simulink model "BallAndPlate_system"  (R2024a)
settings: Solver=ode23t  StartTime=0.0  StopTime=StopTime  RelTol=1e-3  AbsTol=1e-3
settings Model: DataDictionary=BallAndPlate_system_data.sldd  Creator=tshintai  LastModifiedBy=tshintai
settings SolverCC: AutoScaleAbsTol=off  DaesscMode=Fast
settings OptimizationCC: DefaultParameterBehavior=Inlined  EnhancedBackFolding=on  PassReuseOutputArgsAs=Individual arguments  ZeroExternalMemoryAtStartup=off  ZeroInternalMemoryAtStartup=off  OptimizeBlockOrder=speed  DifferentSizesBufferReuse=on  OptimizationCustomize=off  EfficientTunableParamExpr=on
settings DebuggingCC: ParameterPrecisionLossMsg=none  ParameterTunabilityLossMsg=error  UnconnectedInputMsg=warning  UnconnectedOutputMsg=warning  UnconnectedLineMsg=warning
settings ModelReferenceCC: EnableRefExpFcnMdlSchedulingChecks=on
settings SFSimCC: MATLABDynamicMemAlloc=off
settings RTWCC: Description=Embedded Coder  SystemTargetFile=ert.tlc  TemplateMakefile=ert_default_tmf  CodeExecutionProfiling=on  CodeProfilingSaveOptions=AllData  GPUComputeCapability=3.5  DLArmComputeVersion=19.05
settings CodeAppCC: ForceParamTrailComments=on  IgnoreCustomStorageClasses=off  OperatorAnnotations=on  SimulinkDataObjDesc=on  SFDataObjDesc=on  InsertBlockDesc=on
settings ERTTargetCC: TargetLangStandard=C99 (ISO)  GenerateSampleERTMain=on  InlinedParameterPlacement=NonHierarchical  ERTCustomFileTemplate=example_file_process.tlc
settings ExplorerConfigSet: InternalSimMechanicsExplorerSettings="<ExplorerConfiguration><canonicalview>default</canonicalview><AnimationSetting><BasePlaybackSpeed>1.0</BasePlaybackSpeed><PlaybackSpeedFactor>1.0</PlaybackSpeedFactor></AnimationSetting><TilePanel><TileInfo><Tiles Columns=\"1\" Count=\"1\" Rows=\"1\"><Column Weight=\"1\"/><Row Weight=\"1\"/><Tile Height=\"1\" Width=\"1\" X=\"0\" Y=\"0\"/></Tiles></TileInfo><SceneInfo><SceneViewer><BGColor><R>0.60000002384185791</R><G>0.60000002384185791</G><B>0.60000002384185791</B></BGColor><Camera><DoPerspective>on</DoPerspective><Position><X>-0.179931604694393593</X><Y>-0.313436002294735339</Y><Z>0.218441760007596908</Z></Position><Center><X>-0.0553904340360055342</X><Y>-0.0935298101114326597</Y><Z>-0.00250039830421483478</Z></Center><Up><X>0.29243903801469856</X><Y>0.590284090195823952</Y><Z>0.752359024606421567</Z></Up><ViewLimDist>1</ViewLimDist><YLim>0.466307658154998583</YLim><XLim>0.700291216161599284</XLim></Camera></SceneViewer></SceneInfo></TilePanel><MechEditorPanel><Cameras><Camera><Id>Camera1</Id><Value><Name>Camera1</Name><NativeCamera><PositionKeyframeSet><Keyframe><Time>0</Time><Value><X>-0.17993160469439359</X><Y>-0.31343600229473534</Y><Z>0.21844176000759691</Z></Value></Keyframe></PositionKeyframeSet><CenterKeyframeSet><Keyframe><Time>0</Time><Value><X>-0.055390434036005534</X><Y>-0.09352981011143266</Y><Z>-0.0025003983042148348</Z></Value></Keyframe></CenterKeyframeSet><UpVectorKeyframeSet><Keyframe><Time>0</Time><Value><X>0.29243903801469856</X><Y>0.59028409019582395</Y><Z>0.75235902460642157</Z></Value></Keyframe></UpVectorKeyframeSet></NativeCamera></Value></Camera></Cameras><GfxPanelCameraMap><MapElement CameraMLId=\"Camera1\" GfxPanelIndex=\"0\"/></GfxPanelCameraMap><VideoCreator><PlaybackSpeedRatio>1.0</PlaybackSpeedRatio><FrameRate>30</FrameRate><VideoFormat>Motion JPEG AVI</VideoFormat><FrameSize>auto</FrameSize></VideoCreator></MechEditorPanel></ExplorerConfiguration>"

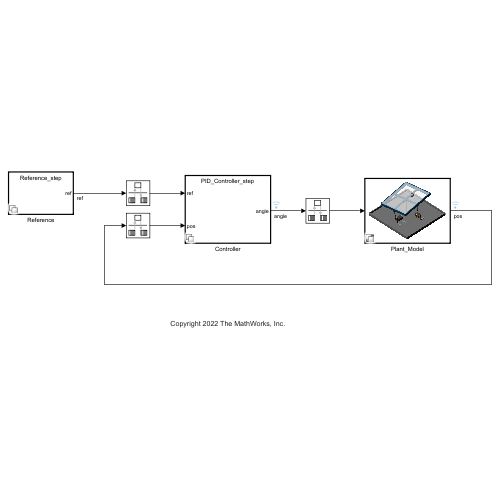
[thumbnail: Simulink's stored preview of the top-level diagram]
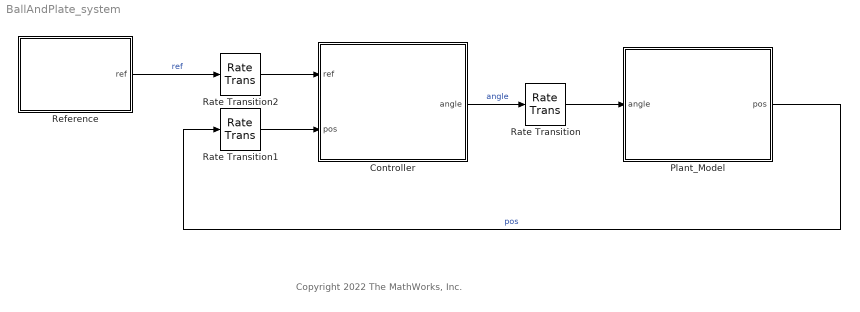
== system BallAndPlate_system ==
  note: Copyright 2022 The MathWorks, Inc.
  Controller : Subsystem  Variant=on  VariantActivationTime=inherit from Simulink.VariantControl
  Plant_Model : Subsystem  Variant=on  VariantActivationTime=inherit from Simulink.VariantControl  PropagateVariantConditions=on
  Rate Transition : RateTransition
  Rate Transition1 : RateTransition  OutPortSampleTime=V_TimeStep
  Rate Transition2 : RateTransition  OutPortSampleTime=V_TimeStep
  Reference : Subsystem  Variant=on  VariantControl=Choice  VariantActivationTime=inherit from Simulink.VariantControl
  wires:
  Plant_Model/1(pos) -> Rate Transition1/1  "pos"
  Controller/1(angle) -> Rate Transition/1  "angle"
  Rate Transition/1 -> Plant_Model/1(angle)
  Rate Transition1/1 -> Controller/2(pos)
  Rate Transition2/1 -> Controller/1(ref)
  Reference/1(ref) -> Rate Transition2/1  "ref"

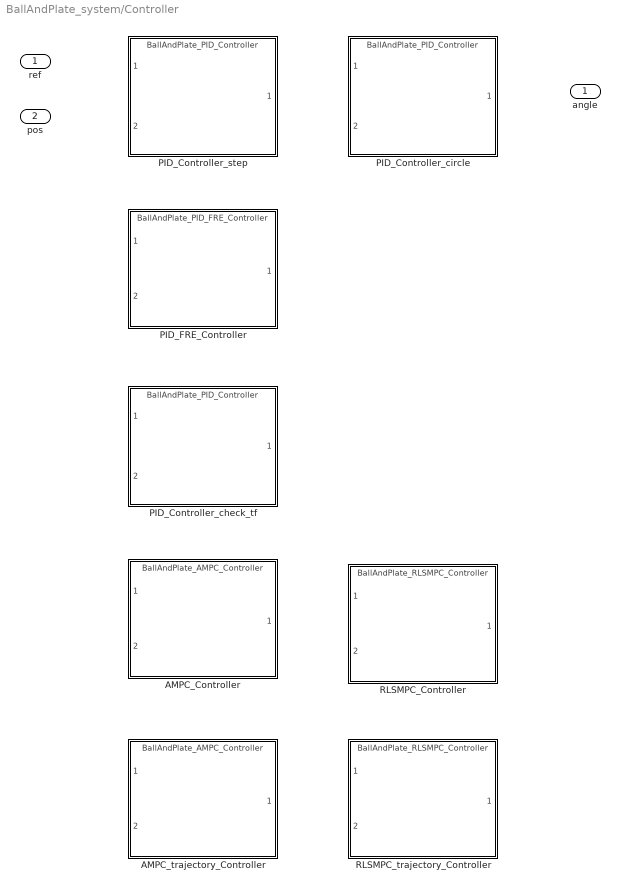
== system BallAndPlate_system/Controller ==
  ref : Inport
  pos : Inport  Port=2
  AMPC_Controller : ModelReference  ModelNameDialog=BallAndPlate_AMPC_Controller.slx  SimulationMode=Normal  VariantControl=SIMMODE_MPC_A  ModelReferenceVersion=6.0
  AMPC_trajectory_Controller : ModelReference  ModelNameDialog=BallAndPlate_AMPC_Controller.slx  SimulationMode=Normal  VariantControl=SIMMODE_MPC_A_TR  ModelReferenceVersion=6.0
  PID_Controller_check_tf : ModelReference  ModelNameDialog=BallAndPlate_PID_Controller  SimulationMode=Normal  VariantControl=SIMMODE_PID_CHECK_TF  ModelReferenceVersion=6.0
  PID_Controller_circle : ModelReference  ModelNameDialog=BallAndPlate_PID_Controller  SimulationMode=Normal  VariantControl=SIMMODE_PID_CIRCLE  ModelReferenceVersion=6.0
  PID_Controller_step : ModelReference  ModelNameDialog=BallAndPlate_PID_Controller  SimulationMode=Normal  VariantControl=SIMMODE_PID_STEP  ModelReferenceVersion=6.0
  PID_FRE_Controller : ModelReference  ModelNameDialog=BallAndPlate_PID_FRE_Controller  SimulationMode=Normal  VariantControl=SIMMODE_PID_FRE  ModelReferenceVersion=6.0
  RLSMPC_Controller : ModelReference  ModelNameDialog=BallAndPlate_RLSMPC_Controller.slx  SimulationMode=Normal  VariantControl=SIMMODE_MPC_ARLS  ModelReferenceVersion=6.0
  RLSMPC_trajectory_Controller : ModelReference  ModelNameDialog=BallAndPlate_RLSMPC_Controller.slx  SimulationMode=Normal  VariantControl=SIMMODE_MPC_ARLS_TR  ModelReferenceVersion=6.0
  angle : Outport

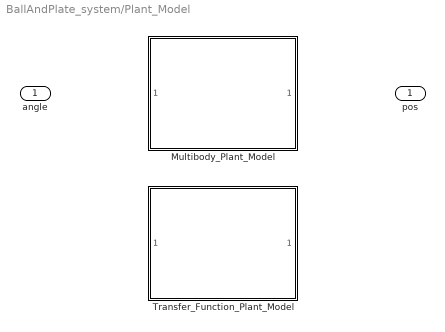
== system BallAndPlate_system/Plant_Model ==
  angle : Inport
  Multibody_Plant_Model : Subsystem  VariantControl=(default)  ReferencedSubsystem=BallAndPlate_plant_model
  Transfer_Function_Plant_Model : Subsystem  VariantControl=SIMMODE_PID_CHECK_TF  ReferencedSubsystem=BallAndPlate_transfer_function_model
  pos : Outport

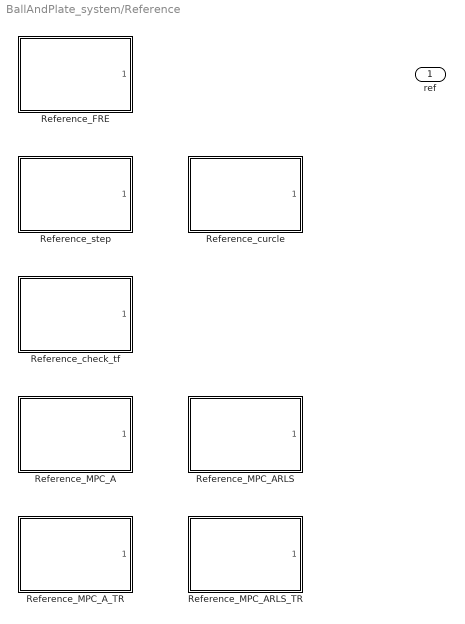
== system BallAndPlate_system/Reference ==
  Reference_FRE : Subsystem  VariantControl=SIMMODE_PID_FRE  ReferencedSubsystem=Reference_stay
  Reference_MPC_A : Subsystem  VariantControl=SIMMODE_MPC_A  ReferencedSubsystem=Reference_step
  Reference_MPC_ARLS : Subsystem  VariantControl=SIMMODE_MPC_ARLS  ReferencedSubsystem=Reference_step
  Reference_MPC_ARLS_TR : Subsystem  VariantControl=SIMMODE_MPC_ARLS_TR  ReferencedSubsystem=Reference_curcle_trajectory
  Reference_MPC_A_TR : Subsystem  VariantControl=SIMMODE_MPC_A_TR  ReferencedSubsystem=Reference_curcle_trajectory
  Reference_check_tf : Subsystem  VariantControl=SIMMODE_PID_CHECK_TF  ReferencedSubsystem=Reference_step
  Reference_curcle : Subsystem  VariantControl=SIMMODE_PID_CIRCLE  ReferencedSubsystem=Reference_curcle
  Reference_step : Subsystem  VariantControl=SIMMODE_PID_STEP  ReferencedSubsystem=Reference_step
  ref : Outport
